simulink model "power_battery_aging_3y"  (R2020b)
settings: Solver=ode23tb  StartTime=0.0  StopTime=3600*24  RelTol=1e-3  EnableMultiTasking=on
undefined symbols (not defined in the file): Ion, Lithium
libraries: electricdrivelib x2, powerlib x2, powerlib_meascontrol x2
settings Model: Creator=MathWorks  LastModifiedBy=qinle
settings DataIOCC: LimitDataPoints=on  ReturnWorkspaceOutputs=off
settings OptimizationCC: LifeSpan=inf
settings DebuggingCC: AllowSymbolicDim=off  SFUnexpectedBacktrackingDiag=warning  SFNoUnconditionalDefaultTransitionDiag=warning  SFExecutionAtInitializationDiag=none  ArithmeticOperatorsInVariantConditions=warning
settings HardwareCC: ProdBitPerPointer=32  ProdBitPerSizeT=32  ProdBitPerPtrDiffT=32  ProdLargestAtomicFloat=None  ProdIntDivRoundTo=Undefined  ProdEndianess=Unspecified  ProdWordSize=32  ProdHWDeviceType=32-bit Generic
settings ModelReferenceCC: PropagateSignalLabelsOutOfModel=off
settings SFSimCC: SimUseLocalCustomCode=off  CustomCodeUndefinedFunction=UseInterfaceOnly
settings RTWCC: RTWUseLocalCustomCode=off
settings CodeAppCC: StateflowObjectComments=on
settings GRTTargetCC: TargetLangStandard=C89/C90 (ANSI)
settings ConfigComp: CovMetricSettings=dw  CovSaveCumulativeToWorkspaceVar=on  CovSaveSingleToWorkspaceVar=on  CovExternalEMLEnable=off
settings SimscapeCC: SimscapeNormalizeSystem=off

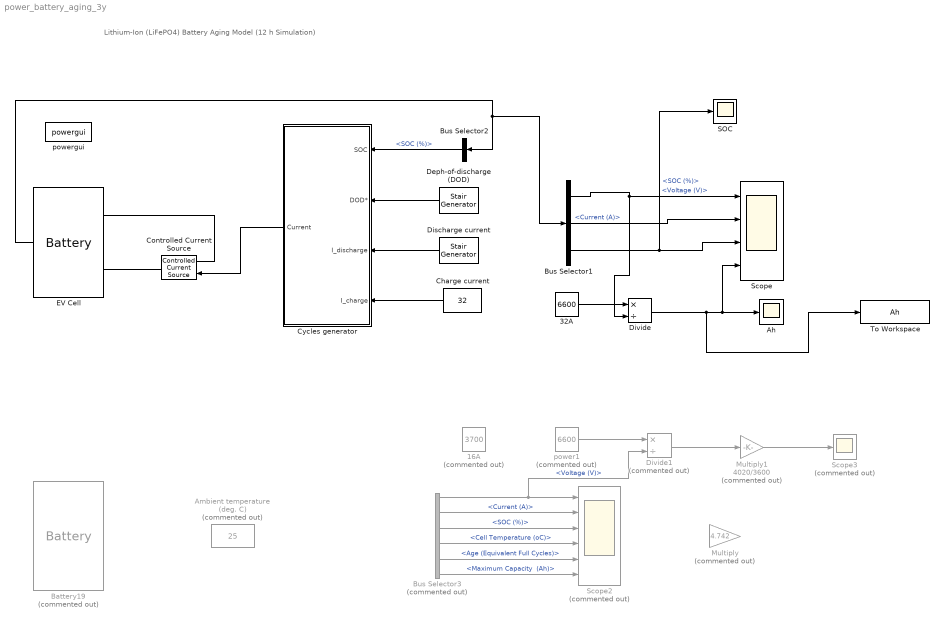
== system power_battery_aging_3y ==
  note: Lithium-Ion (LiFePO4) Battery Aging Model (12 h Simulation)
  16A : Constant  Commented=on  Value=3700
  32A : Constant  Value=6600
  Ah : Scope
  Ambient temperature (deg. C) : Constant  Commented=on  Value=25
  Battery19 : electricdrivelib/Extra Sources/Battery  Commented=on  BatType=Lithium-Ion  ShowTempParam=on  ThermalPreset="12.8V  40Ah  (LiFeMgPO4)"  ShowAgeParam=on  NomV=12.6  NomQ=40  SOC=10  Batt_Tr=90  PresetModel=off  MaxQ=40  MinV=10.5  FullV=13.8  Dis_rate=20  R=0.015  Normal_OP=30.14  expZone="[13.1          0.5]"  current=[0.15 1.3 3.25]  Units=Ampere-hour  Tci=25  NomT=20  T2=0  MaxQ2=36  FullV2=13  Normal_OP2=11.7  expZone2="[12.67            4]"  Rca=0.6411  ti=4880  Dp=0  Neq0=0  Tsim=30  Ta1=23  Qeol=40*0.9  Reol=0.0126*1.2  Char_age=[20, 26]  Dis_age=[20, 80]  N1=1500  N2=10445  N3=1017  N4=1460  Ta2=45  N5=982
  Bus Selector1 : BusSelector  OutputSignals=Voltage (V),Current (A),SOC (%)
  Bus Selector2 : BusSelector  OutputSignals=SOC (%)
  Bus Selector3 : BusSelector  Commented=on  OutputSignals="Voltage (V),Current (A),SOC (%),Cell Temperature (oC),Age (Equivalent Full Cycles),Maximum Capacity  (Ah)"
  Charge current : Constant  Value=32
  Controlled Current Source : powerlib/Electrical Sources/Controlled Current Source  Initialize=on  Source_Type=AC  Amplitude=0  Phase=0  Frequency=0  Measurements=None
  Cycles generator : Subsystem
  Deph-of-discharge (DOD) : powerlib_meascontrol/Pulse & Signal Generators/Stair Generator  t=[0 50 100]*14400  e=[20 80 20]  Ts=0
  Discharge current : powerlib_meascontrol/Pulse & Signal Generators/Stair Generator  t=[0 150 200]*14400  e=[1 4 1]*20  Ts=0
  Divide : Product  Inputs=*/
  Divide1 : Product  Commented=on  Inputs=*/
  EV Cell : electricdrivelib/Extra Sources/Battery  BatType=Lithium-Ion  ShowTempParam=off  ThermalPreset="12.8V  40Ah  (LiFeMgPO4)"  ShowAgeParam=on  NomV=230  NomQ=170  SOC=10  Batt_Tr=90  PresetModel=on  MaxQ=170  MinV=172.5  FullV=267.717  Dis_rate=73.913  R=0.013529  Normal_OP=153.7391  expZone="[248.4887      8.352174]"  current=[0.15 1.3 3.25]  Units=Ampere-hour  Tci=25  NomT=20  T2=0  MaxQ2=36  FullV2=13  Normal_OP2=11.7  expZone2="[12.67            4]"  Rca=0.6411  ti=4880  Dp=0  Neq0=0  Tsim=30  Ta1=23  Qeol=40*0.9  Reol=0.0126*1.2  Char_age=[20, 26]  Dis_age=[20, 80]  N1=1500  N2=10445  N3=1017  N4=1460  Ta2=45  N5=982
  Multiply : Gain  Commented=on  Gain=4.742
  Multiply1 : Gain  Commented=on  Gain=4020/3600
  SOC : Scope
  Scope : Scope  NumInputPorts=4
  Scope2 : Scope  Commented=on  NumInputPorts=6
  Scope3 : Scope  Commented=on
  To Workspace : ToWorkspace  VariableName=Ah  SampleTime=900
      settings: Save2DSignal=2-D array (concatenate along first dimension)
  power1 : Constant  Commented=on  Value=6600
  powergui : powerlib/powergui  SimulationMode=Continuous  SampleTime=0.001  frequency=60  Iterations=50  frequencyindice=0  Pbase=100e6  ErrMax=1e-4  UnitsV=kV  UnitsW=MW  buscounter=0  FunctionMessages=off  echomessages=off  EnableUseOfTLC=off  CurrentSourceSwitches=on  DisableSnubberDevices=off  DisableRonSwitches=off  DisableVfSwitches=off  DisplayEquations=off  AutomaticDiscreteSolvers=off  SolverType=Tustin  Interpol=off  ExternalGateDelay=off  methode=off  Ts=0  x0status=blocks  SPID=off  SwTol=0  HookPort=off  NonlinearTolerance=1e-4  nMaxIteration=100  ContinueOnMaxIteration=off  RestoreLinks=warning  ResistiveCurrentMeasurement=off  Frange=[0:2:500]  Ylog=off  Xlog=on  ShowGrid=off  save=off  variable=ZData  structure=0  ZoomFFT=on  StartTime=0.0  cycles=1  DisplayStyle=1  fundamental=60  FreqAxis=off  MaxFrequency=1000  frequencyindicesteady=1  RmsSteady=1  display=off
  wires:
  Bus Selector1/1 -> Divide/2, Scope/1  "<Voltage (V)>"
  Bus Selector1/2 -> Scope/2  "<Current (A)>"
  Bus Selector1/3 -> SOC/1, Scope/3  "<SOC (%)>"
  Cycles generator/1(Current) -> Controlled Current Source/1
  Bus Selector2/1 -> Cycles generator/1(SOC)  "<SOC (%)>"
  Charge current/1 -> Cycles generator/4(I_charge)
  Deph-of-discharge (DOD)/1 -> Cycles generator/2(DOD*)
  Discharge current/1 -> Cycles generator/3(I_discharge)
  32A/1 -> Divide/1
  Divide1/1 -> Multiply1/1
  power1/1 -> Divide1/1
  Bus Selector3/1 -> Divide1/2, Scope2/1  "<Voltage (V)>"
  Bus Selector3/5 -> Scope2/5  "<Age (Equivalent Full Cycles)>"
  Bus Selector3/3 -> Scope2/3  "<SOC (%)>"
  Bus Selector3/2 -> Scope2/2  "<Current (A)>"
  Bus Selector3/4 -> Scope2/4  "<Cell Temperature (oC)>"
  Bus Selector3/6 -> Scope2/6  "<Maximum Capacity  (Ah)>"
  Multiply1/1 -> Scope3/1
  Divide/1 -> Ah/1, Scope/4, To Workspace/1
  EV Cell/1 -> Bus Selector2/1, Bus Selector1/1
  connections:
  Controlled Current Source/RConn1 -- EV Cell/LConn2
  Controlled Current Source/LConn1 -- EV Cell/LConn1

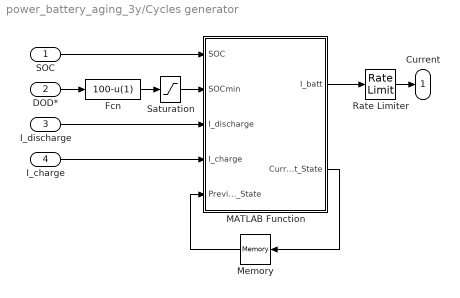
== system power_battery_aging_3y/Cycles generator ==
  SOC : Inport
  DOD* : Inport  Port=2
  I_discharge : Inport  Port=3
  I_charge : Inport  Port=4
  Fcn : Fcn  Expr=100-u(1)
  MATLAB Function : MATLAB Function  TreatAsAtomicUnit=on
  Memory : Memory  InitialCondition=1
  Rate Limiter : RateLimiter  RisingSlewLimit=1000  FallingSlewLimit=-1000  SampleTimeMode=inherited
  Saturation : Saturate  UpperLimit=98  LowerLimit=1
  Current : Outport  VectorParamsAs1DForOutWhenUnconnected=off
  wires:
  MATLAB Function/1(I_batt) -> Rate Limiter/1
  SOC/1 -> MATLAB Function/1(SOC)
  Memory/1 -> MATLAB Function/5(Previous_State)
  MATLAB Function/2(Current_State) -> Memory/1
  DOD*/1 -> Fcn/1
  Fcn/1 -> Saturation/1
  Saturation/1 -> MATLAB Function/2(SOCmin)
  I_discharge/1 -> MATLAB Function/3(I_discharge)
  I_charge/1 -> MATLAB Function/4(I_charge)
  Rate Limiter/1 -> Current/1

== matlab function power_battery_aging_3y/Cycles generator/MATLAB Function ==
  data: SOC input; SOCmin input; I_discharge input; I_charge input; I_batt output; Previous_State input; Current_State output
function [I_batt,Current_State] = fcn(SOC,SOCmin,I_discharge,I_charge,Previous_State)
%cycle generator
Current_State=Previous_State;
if(Previous_State==0 && SOC>=79)
    Current_State=1;
end
if(Previous_State==1 && SOC<=SOCmin)
    Current_State=0;
end
if (Previous_State==1)
    I_batt=I_discharge;
else
    I_batt=-I_charge;
end
